simulink model "MagnetoShield_LQ_MEGA_SISO"  (R2019a)
settings: Solver=FixedStepAuto  StartTime=0.0  StopTime=20  RelTol=1e-3  EnableMultiTasking=on
undefined symbols (not defined in the file): A, B, C, D, DiscIntNeverNeededParam, Discrete, i0, K, MEGA, R, Time, Ts, u0, UNO, y0
libraries: MagnetoLibrary x2, ctrlSharedLib x1, CommonBlocks x1
settings Model: SimulationMode=external  ExtModeTrigDuration=2  Creator=Jakub  LastModifiedBy=jakub
settings OptimizationCC: EnhancedBackFolding=on  PassReuseOutputArgsAs=Individual arguments  MaxStackSize=64  OptimizeBlockOrder=speed  DifferentSizesBufferReuse=on  OptimizationCustomize=off
settings DebuggingCC: ParameterTunabilityLossMsg=error
settings HardwareCC: ProdBitPerInt=16  ProdBitPerPointer=16  ProdBitPerSizeT=16  ProdBitPerPtrDiffT=16  ProdLargestAtomicFloat=None  ProdWordSize=8  ProdHWDeviceType=Atmel->AVR
settings SFSimCC: MATLABDynamicMemAlloc=off
settings RTWCC: SystemTargetFile=ert.tlc  HardwareBoard=Arduino Mega 2560  TLCOptions=-aInlineSetEventsForThisBaseRateFcn=TLC_FALSE -aSuppressMultiTaskScheduler=TLC_FALSE -aRateBasedStepFcn=1  TemplateMakefile=ert_default_tmf  GenerateReport=on  Toolchain=Arduino AVR  BuildConfiguration=Faster Runs  IncludeHyperlinkInReport=on  LaunchReport=on  GenerateTraceInfo=on  GenerateTraceReport=on  GenerateTraceReportSl=on  GenerateTraceReportSf=on  GenerateTraceReportEml=on
settings CodeAppCC: ForceParamTrailComments=on  IgnoreCustomStorageClasses=off  OperatorAnnotations=on  SimulinkDataObjDesc=on  SFDataObjDesc=on  InsertBlockDesc=on
settings ERTTargetCC: SupportContinuousTime=on  SupportVariableSizeSignals=on  ExtModeStaticAllocSize=2048

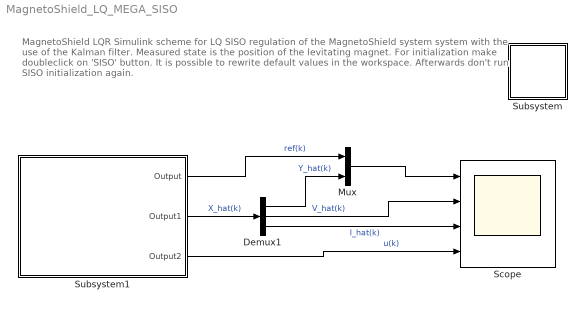
== system MagnetoShield_LQ_MEGA_SISO ==
  note: MagnetoShield LQR
      | Simulink scheme for LQ SISO regulation of the MagnetoShield system system with the use of
      | the Kalman filter. Measured state is the position of the levitating magnet. For initialization make
      | doubleclick on 'SISO' button.
      | It is possible to rewrite default values in the workspace. Afterwards don't run SISO initialization again.
  Demux1 : Demux  Outputs=3
  Mux : Mux  Inputs=2
  Scope : Scope  NumInputPorts=4
  Subsystem : Subsystem
      settings: OpenFcn=|
      | clear;close all;clc;
      | cd(fileparts(which(gcs)));
      | load '../../../../matlab/examples/MagnetoShield/MagnetoShield_Models_Greybox_SS';
      | %% MagnetoShield - LQR simulation and control initialization for Simulink
      | 
      | order = 'SISO';                 % SISO - position / SIMO - position & current
      | Ts = 0.0025;                    % Sampling of the Simulink simulation
      | 
      | % Matrices extraction from model
      | modeld=c2d(model,Ts);           % Discretized linear state-space model
      | A = modeld.a;                   % Extract A
      | B = modeld.b;                   % Extract B
      | Ci = [1 0 0];                   % Position is measured for integrator 'xi' computation
      | D = 0;
      | 
      | % Discrete augmented model with integrator state - unstable, unobservable
      | Ai = [1 -Ci;
      |       zeros(3,1) A];
      | Bi = [0;B];
      | 
      | % LQ gain computation - the 1. tuning diverges in the simulations but is
      | % smoother in experiments:
      | %Experiments
      | Qlq=diag([30 180 120 60]);      % State penalty matrix
      | Rlq=0.0001;                       % Input penalty matrix
      | K=dlqr(Ai,Bi,Qlq,Rlq);         % LQ gain for system states
      | 
      | % Measurement matrices of state-space and Kalman filter gains
      | if order == 'SISO'                  % Setup if just position is measured
      |     C = [1 0 0];
      |     D = 0;
      |     Q = diag([0.0001, 100, 100]);   % Penalty of the model for Kalman filter
      |     R = 0.001;                     % Penalty of measurement for Kalman filter
      | 
      | elseif order == 'SIMO'             % Setup if position and current are measured
      |     C = [1 0 0;0 0 1];
      |     D = [0;0];
      |     Q = diag([0.0001, 100, 80]);   % Penalty of the model for Kalman filter
      |     R = [0.001, 0.01];             % Penalty of measurement for Kalman filter
      | end
      mask Display: disp('SISO')
  Subsystem1 : Subsystem
  wires:
  Demux1/2 -> Scope/2  "V_hat(k)"
  Demux1/3 -> Scope/3  "I_hat(k)"
  Subsystem1/2(Output1) -> Demux1/1  "X_hat(k)"
  Demux1/1 -> Mux/2  "Y_hat(k)"
  Mux/1 -> Scope/1
  Subsystem1/1(Output) -> Mux/1  "ref(k)"
  Subsystem1/3(Output2) -> Scope/4  "u(k)"

== system MagnetoShield_LQ_MEGA_SISO/Subsystem ==

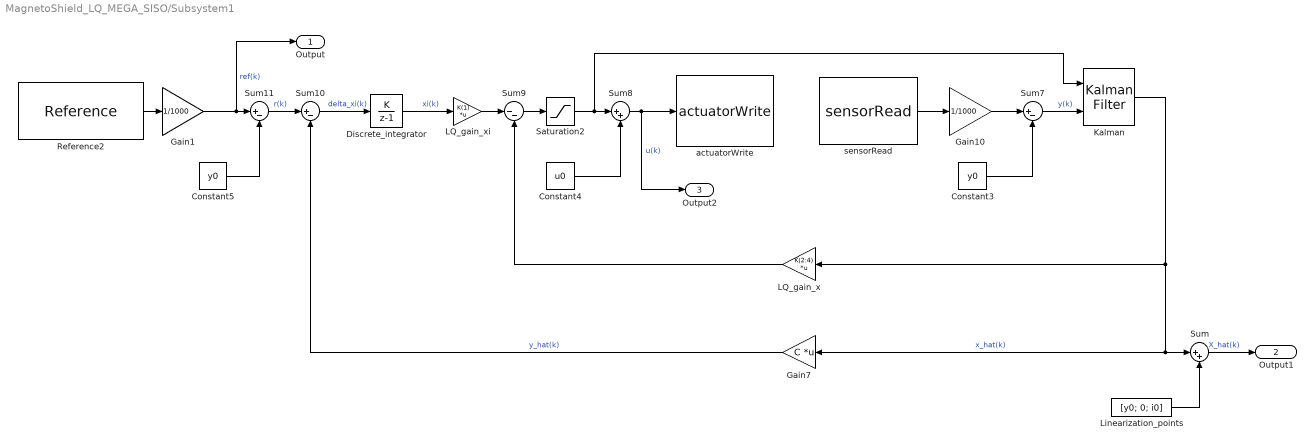
== system MagnetoShield_LQ_MEGA_SISO/Subsystem1 ==
  Constant3 : Constant  Value=y0
  Constant4 : Constant  Value=u0  SampleTime=Ts
  Constant5 : Constant  Value=y0
  Discrete_integrator : DiscreteIntegrator  IntegratorMethod=Accumulation: Forward Euler  SampleTime=Ts  LimitOutput=on  UpperSaturationLimit=1  LowerSaturationLimit=-1  ICPrevOutput=DiscIntNeverNeededParam  ICPrevScaledInput=DiscIntNeverNeededParam
  Gain1 : Gain  Gain=1/1000
  Gain10 : Gain  Gain=1/1000
  Gain7 : Gain  Gain=C  Multiplication=Matrix(K*u)
  Kalman : ctrlSharedLib/Kalman Filter  TimeDomain=Discrete-Time  UseCurrentEstimator=on  ModelSource=Individual A, B, C, D matrices  ModelSourceVariable=ss(0.95,1,1,0,1)  A=A  B=B  C=C  D=D  NumberOfStates=1  NumberOfInputs=1  NumberOfOutputs=1  InitialEstimateSource=Dialog  X0=0  P0=10  UseK=off  UseGH=off  NumberOfProcessNoiseInputs=1  G=1  TimeInvariantG=on  H=0  TimeInvariantH=on  Q=Q  TimeInvariantQ=on  R=R  TimeInvariantR=on  N=0  TimeInvariantN=on  AddInputPort=on  AddEnablePort=off  OutputEstimatedY=off  OutputP=off  Ts=-1
  LQ_gain_x : Gain  Gain=K(2:4)  Multiplication=Matrix(K*u)
  LQ_gain_xi : Gain  Gain=K(1)  Multiplication=Matrix(K*u)
  Linearization_points : Constant  Value=[y0; 0; i0]
  Reference2 : CommonBlocks/Reference  RefVect=[15, 13, 16, 14.5,16.5,12.5,15,17]  AtTheEnd=Stop simulation  Reps=5  SectLen=1000  OffsetTime=0  Ts=Ts
      settings: SourceProductName=AutomationShield
  Saturation2 : Saturate  UpperLimit=10-u0  LowerLimit=0-u0
  Sum : Sum  Inputs=|++
  Sum10 : Sum  Inputs=|+-
  Sum11 : Sum  Inputs=|+-
  Sum7 : Sum  Inputs=|+-
  Sum8 : Sum  Inputs=|++
  Sum9 : Sum  Inputs=|--
  actuatorWrite : MagnetoLibrary/actuatorWrite  Board=UNO/MEGA  Units=Volts
      settings: SourceProductName=AutomationShield
  sensorRead : MagnetoLibrary/sensorRead  board=UNO/MEGA  sensor=Distance [mm]  sampling=Ts
      settings: SourceProductName=AutomationShield
  Output : Outport
  Output1 : Outport  Port=2
  Output2 : Outport  Port=3
  wires:
  Gain1/1 -> Output/1, Sum11/1  "ref(k)"
  Kalman/1 -> Sum/1, Gain7/1, LQ_gain_x/1  "x_hat(k)"
  Gain10/1 -> Sum7/1
  Discrete_integrator/1 -> LQ_gain_xi/1  "xi(k)"
  sensorRead/1 -> Gain10/1
  Sum8/1 -> Output2/1, actuatorWrite/1  "u(k)"
  Sum9/1 -> Saturation2/1
  Constant3/1 -> Sum7/2
  Sum11/1 -> Sum10/1  "r(k)"
  LQ_gain_x/1 -> Sum9/2
  Saturation2/1 -> Kalman/1, Sum8/1
  LQ_gain_xi/1 -> Sum9/1
  Sum10/1 -> Discrete_integrator/1  "delta_xi(k)"
  Sum7/1 -> Kalman/2  "y(k)"
  Linearization_points/1 -> Sum/2
  Reference2/1 -> Gain1/1
  Gain7/1 -> Sum10/2  "y_hat(k)"
  Constant5/1 -> Sum11/2
  Constant4/1 -> Sum8/2
  Sum/1 -> Output1/1  "X_hat(k)"
